simulink model "Carrier_Phase_Shift"  (R2021a)
settings: Solver=FixedStepAuto  StartTime=0.0  StopTime=0.05  FixedStep=1e-7  MaxStep=1e-7  RelTol=1e-6
InitFcn:
  | fsw=50e3;
  | ma=0.6;
  | ffund=100;
  | 
  | L1=63e-6;
  | L2=50e-6;
  | M=18e-6;
  | C1=12.2e-9;
  | C2=14.5e-9;
  | R=20;
  | 
  | sn3=C1*C2*M*R;
  | sd4=C1*C2*L1*L2+C1*C2*L1*M+C1*C2*L2*M;
  | sd3= C1*C2*L1*R+ C1*C2*M*R;
  | sd2= C1*L1+C2*L2+C1*M+C2*M;
  | sd1=C2*R;
  | sd0=1;
libraries: spsSeriesRLCBranchLib x9, spsDiodeLib x4, spsVoltageMeasurementLib x3, spsControlledVoltageSourceLib x1, spsCurrentMeasurementLib x1, dspsigops x1, spspowerguiLib x1
settings Model: Creator=enes_  LastModifiedBy=enes_
settings DataIOCC: SaveFormat=StructureWithTime  ReturnWorkspaceOutputs=off

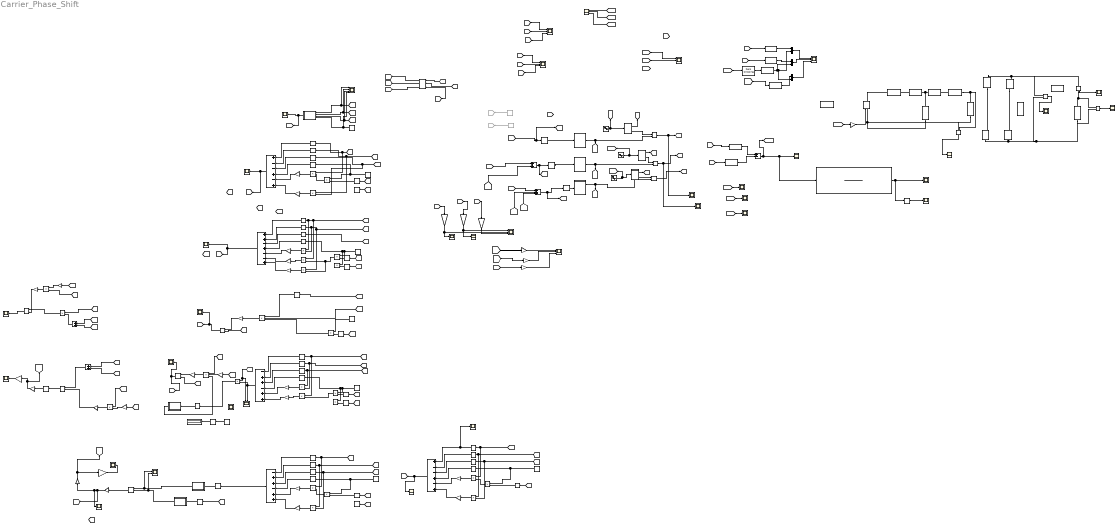
== system Carrier_Phase_Shift ==
  Abs : Abs
  Add : Sum  Inputs=+--+-+
  Add1 : Sum  Inputs=++-+--+
  Add2 : Sum  Inputs=-++-++
  Add3 : Sum
  Add4 : Sum
  Add5 : Sum
  Add6 : Sum  Inputs=+--+-+
  Add7 : Sum  Inputs=+++
  Add8 : Sum  Inputs=-++-++
  Atan : Trigonometry  Operator=atan
  Atan1 : Trigonometry  Operator=atan2
  Constant : Constant  Commented=on  Value=0
  Constant{1,3..8} (7 alike) : Constant  Value=0.95
  Constant2 : Constant  Commented=on  Value=pi
  Controlled Voltage Source : spsControlledVoltageSourceLib/Controlled Voltage Source  Initialize=on  Source_Type=AC  Amplitude=0  Phase=0  Frequency=0  Measurements=None
  Cos{,2,4,8..9} (5 alike) : Trigonometry  Operator=cos
  Cos{1,3,5..6,10} (5 alike) : Trigonometry
  Current Measurement : spsCurrentMeasurementLib/Current Measurement  PhasorSimulation=off  OutputType=Complex  PSBequivalent=0
  Data Type Conversion{,1..2,4..6} (6 alike) : DataTypeConversion
  Delay : Delay  DelayLength=1
  Delay1 : Delay  DelayLength=1
  Delay2 : Delay  DelayLength=1
  Diode{,1..3} (4 alike) : spsDiodeLib/Diode  Ron=0.001  Lon=0  Vf=0.8  IC=0  UseSnubber=0  Rs=500  Cs=250e-9  Measurements=on
  Display : Display
  Divide{,1,3..4} (4 alike) : Product  Inputs=*/
  Gain : Gain  Gain=100
  Gain10 : Gain  Gain=8
  Gain{9,12..13,23,28..30,33} (8 alike) : Gain  Gain=180/pi
  Gain{2..3,5..7,14..16,18,20,22,25,27,31..32,34} (16 alike) : Gain  Gain=2
  Gain17 : Gain  Gain=4
  Gain19 : Gain  Gain=4
  Gain21 : Gain  Gain=4
  Gain35 : Gain  Gain=-1
  Goto18 : Goto  Commented=on  GotoTag=CP_A
  Goto19 : Goto  Commented=on  GotoTag=CP_BA
  MATLAB Function : MATLAB Function  TreatAsAtomicUnit=on
  MATLAB Function1 : MATLAB Function  TreatAsAtomicUnit=on
  MATLAB Function2 : MATLAB Function  TreatAsAtomicUnit=on
  MATLAB Function3 : MATLAB Function  TreatAsAtomicUnit=on
  Mux : Mux  Inputs=2
  Mux1 : Mux  Inputs=2
  Mux2 : Mux  Inputs=2
  Product{,1..7,9..14,16..19,21..23,25..26} (23 alike) : Product
  Product15 : Product  Inputs=3
  Product8 : Product  Inputs=3
  Relational Operator : RelationalOperator  OutDataTypeStr=boolean  RndMeth=Simplest
  Relational Operator1 : RelationalOperator  OutDataTypeStr=boolean  RndMeth=Simplest
  Relational Operator2 : RelationalOperator  OutDataTypeStr=boolean  RndMeth=Simplest
  Scope{,8,27,29..30,38..39} (7 alike) : Scope  NumInputPorts=3
  Scope{1..7,9..14,16..22,25..26,28,31,33} (25 alike) : Scope
  Scope15 : Scope  NumInputPorts=4
  Scope23 : Scope  NumInputPorts=2
  Scope24 : Scope  NumInputPorts=2
  Scope32 : Scope  NumInputPorts=2
  Series RLC Branch : spsSeriesRLCBranchLib/Series RLC Branch  LConnTagsString=__new0  RConnTagsString=__new0  BranchType=C  Resistance=1  Inductance=1e-3  SetiL0=off  InitialCurrent=0  Capacitance=12.2e-9  Setx0=off  InitialVoltage=0  Measurements=None
  Series RLC Branch1 : spsSeriesRLCBranchLib/Series RLC Branch  LConnTagsString=__new0  RConnTagsString=__new0  BranchType=C  Resistance=1  Inductance=1e-3  SetiL0=off  InitialCurrent=0  Capacitance=14.5e-9  Setx0=off  InitialVoltage=0  Measurements=None
  Series RLC Branch2 : spsSeriesRLCBranchLib/Series RLC Branch  LConnTagsString=__new0  RConnTagsString=__new0  BranchType=L  Resistance=1  Inductance=63e-6  SetiL0=off  InitialCurrent=0  Capacitance=1e-6  Setx0=off  InitialVoltage=0  Measurements=None
  Series RLC Branch3 : spsSeriesRLCBranchLib/Series RLC Branch  LConnTagsString=__new0  RConnTagsString=__new0  BranchType=L  Resistance=1  Inductance=18e-6  SetiL0=off  InitialCurrent=0  Capacitance=1e-6  Setx0=off  InitialVoltage=0  Measurements=None
  Series RLC Branch4 : spsSeriesRLCBranchLib/Series RLC Branch  LConnTagsString=__new0  RConnTagsString=__new0  BranchType=L  Resistance=1  Inductance=50e-6  SetiL0=off  InitialCurrent=0  Capacitance=1e-6  Setx0=off  InitialVoltage=0  Measurements=None
  Series RLC Branch5 : spsSeriesRLCBranchLib/Series RLC Branch  LConnTagsString=__new0  RConnTagsString=__new0  BranchType=C  Resistance=1  Inductance=1e-3  SetiL0=off  InitialCurrent=0  Capacitance=100e-6  Setx0=off  InitialVoltage=0  Measurements=None
  Series RLC Branch6 : spsSeriesRLCBranchLib/Series RLC Branch  LConnTagsString=__new0  RConnTagsString=__new0  BranchType=L  Resistance=1  Inductance=500e-6  SetiL0=off  InitialCurrent=0  Capacitance=14.5e-9  Setx0=off  InitialVoltage=0  Measurements=None
  Series RLC Branch7 : spsSeriesRLCBranchLib/Series RLC Branch  LConnTagsString=__new0  RConnTagsString=__new0  BranchType=R  Resistance=40  Inductance=5e-3  SetiL0=off  InitialCurrent=0  Capacitance=1e-6  Setx0=off  InitialVoltage=0  Measurements=None
  Series RLC Branch8 : spsSeriesRLCBranchLib/Series RLC Branch  LConnTagsString=__new0  RConnTagsString=__new0  BranchType=R  Resistance=40  Inductance=5e-3  SetiL0=off  InitialCurrent=0  Capacitance=1e-6  Setx0=off  InitialVoltage=0  Measurements=None
  Sine Wave : Sin  Amplitude=ma  Frequency=2*pi*ffund  SampleTime=0
  Sine Wave1 : Sin  Amplitude=ma  Frequency=2*pi*ffund  Phase=2*pi/3  SampleTime=0
  Sine Wave2 : Sin  Amplitude=ma  Frequency=2*pi*ffund  Phase=-2*pi/3  SampleTime=0
  Sqrt{,1..3} (4 alike) : Sqrt  OutputSignalType=real  SaturateOnIntegerOverflow=on
  Square{,1..20} (21 alike) : Math  Operator=square  SaturateOnIntegerOverflow=on
  Subsystem2 : Subsystem
  Subsystem3 : Subsystem
  Subsystem4 : Subsystem
  Subsystem5 : Subsystem
  Subtract : Sum  Inputs=+-
  Transfer Fcn : TransferFcn  Numerator=[sn3 0 0 0]  Denominator=[sd4 sd3 sd2 sd1 sd0]
  Triangle Generator-A : Subsystem
  Triangle Generator-A1 : Subsystem
  Triangle Generator-A2 : Subsystem
  Voltage Measurement : spsVoltageMeasurementLib/Voltage Measurement  PhasorSimulation=off  OutputType=Complex  PSBequivalent=0
  Voltage Measurement1 : spsVoltageMeasurementLib/Voltage Measurement  PhasorSimulation=off  OutputType=Complex  PSBequivalent=0
  Voltage Measurement2 : spsVoltageMeasurementLib/Voltage Measurement  PhasorSimulation=off  OutputType=Complex  PSBequivalent=0
  Zero Crossing2 : dspsigops/Zero Crossing  InputProcessing=Columns as channels (frame based)
      settings: SourceProductBaseCode=DS
  Zero3 : Constant  Value=1e-15  OutDataTypeStr=Inherit: Inherit via back propagation
  powergui : spspowerguiLib/powergui  Priority=1  SimulationMode=Continuous  SampleTime=50e-6  frequency=60  Iterations=50  frequencyindice=0  Pbase=100e6  ErrMax=1e-4  UnitsV=kV  UnitsW=MW  buscounter=0  FunctionMessages=off  echomessages=off  EnableUseOfTLC=off  CurrentSourceSwitches=off  DisableSnubberDevices=off  DisableRonSwitches=off  DisableVfSwitches=off  DisplayEquations=off  AutomaticDiscreteSolvers=off  SolverType=Tustin/Backward Euler (TBE)  Interpol=off  ExternalGateDelay=off  methode=off  Ts=100  x0status=blocks  SPID=on  SwTol=0  HookPort=off  NonlinearTolerance=1e-4  nMaxIteration=100  ContinueOnMaxIteration=off  RestoreLinks=warning  ResistiveCurrentMeasurement=off  Frange=[0:2:500]  Ylog=off  Xlog=on  ShowGrid=off  save=off  variable=ZData  structure=0  ZoomFFT=off  StartTime=0.0  cycles=1  DisplayStyle=1  fundamental=60  FreqAxis=off  MaxFrequency=1000  frequencyindicesteady=1  RmsSteady=1  display=off
  wires:
  Triangle Generator-A2/1(Carrier) -> [C_C], Relational Operator2/2
  Relational Operator1/1 -> Scope7/1, [PWMB]
  Data Type Conversion/1 -> Subtract/1
  Data Type Conversion1/1 -> Subtract/2
  Delay1/1 -> Triangle Generator-A1/1(Phase)
  Delay2/1 -> Triangle Generator-A2/1(Phase)
  Add3/1 -> Delay1/1, [CP_B]
  Subtract/1 -> [PWMAB], Transfer Fcn/1, Scope2/1
  Delay/1 -> Triangle Generator-A/1(Phase)
  Gain12/1 -> Scope17/1, Scope27/1
  Gain13/1 -> Scope16/1, Scope27/2
  Subsystem4/2(Out2) -> Relational Operator2/1
  [DA] -> Scope29/1
  [DB] -> Scope29/2
  [Phase] -> Scope29/3
  [SB] -> Scope30/2
  [Phase] -> Scope30/3
  [SA] -> Scope30/1
  Triangle Generator-A/1(Carrier) -> Relational Operator/2, [C_A]
  Zero Crossing2/1 -> Data Type Conversion6/1
  [alpha] -> Add3/2
  [phi] -> Add3/1
  [CP_B] -> Gain13/1
  [CP_A] -> Gain12/1
  Subsystem2/1(Out1) -> [DA]
  Subsystem2/2(Out2) -> Relational Operator/1
  Triangle Generator-A1/1(Carrier) -> Relational Operator1/2, [C_B]
  Sine Wave1/1 -> [R_B], Subsystem3/1(In1)
  Subsystem3/1(Out1) -> [DB]
  Subsystem3/2(Out2) -> Relational Operator1/1
  Sine Wave/1 -> Subsystem2/1(In1), [R_A]
  [PWMA] -> Data Type Conversion4/1
  Mux/1 -> Scope39/1
  Mux1/1 -> Scope39/2
  Data Type Conversion4/1 -> Mux/1
  [PWMB] -> Data Type Conversion5/1
  Data Type Conversion5/1 -> Mux1/1
  Data Type Conversion6/1 -> Mux1/2, Mux2/2, Mux/2
  Relational Operator/1 -> Scope6/1, [PWMA]
  Relational Operator2/1 -> [PWMC]
  [PWMA] -> Data Type Conversion/1
  [PWMB] -> Data Type Conversion1/1
  [PWMAB] -> Data Type Conversion2/1
  Mux2/1 -> Scope39/3
  Data Type Conversion2/1 -> Mux2/1
  [C_A] -> Zero Crossing2/1
  [C_A] -> Scope/1
  [C_B] -> Scope/2
  [PWMAB] -> Gain/1
  Gain/1 -> Controlled Voltage Source/1
  Voltage Measurement/1 -> Scope1/1
  Voltage Measurement1/1 -> Scope3/1
  Current Measurement/1 -> Scope4/1
  Voltage Measurement2/1 -> Scope5/1
  [R_B] -> Scope38/2
  [R_C] -> Scope38/3
  [R_A] -> Scope38/1
  Constant/1 -> Goto18/1
  Constant2/1 -> Goto19/1
  [C_A] -> Scope9/1
  [C_B] -> Scope10/1
  [C_C] -> Scope11/1
  Transfer Fcn/1 -> Abs/1, Scope12/1
  Abs/1 -> Scope13/1
  Sine Wave2/1 -> [R_C], Subsystem4/1(In1)
  Subsystem4/1(Out1) -> [DC]
  Subsystem5/2(Out2) -> [SB]
  [DA] -> Subsystem5/1(In1)
  [DB] -> Subsystem5/2(In2)
  Subsystem5/1(Out1) -> [SA]
  Subsystem5/3(Out3) -> [SC]
  [DC] -> Subsystem5/3(In3)
  [SB] -> Scope15/2, MATLAB Function/2(SB)
  Constant4/1 -> Scope15/4, MATLAB Function/4(SABC)
  [SA] -> Scope15/1, MATLAB Function/1(SA)
  [SC] -> Scope15/3, MATLAB Function/3(SC)
  [phi] -> [CP_A], Delay/1
  MATLAB Function/1(phi) -> [phi], Scope14/1
  [SC] -> Product2/2, Square2/1
  Constant1/1 -> Product1/1, Square3/1
  [SB] -> Product2/1, Square1/1
  [SA] -> Product/1, Square/1
  [phi] -> Cos/1
  [phi] -> Cos1/1
  Cos/1 -> Product1/2
  Product1/1 -> Product/2
  Product/1 -> Gain2/1
  Product2/1 -> Gain3/1
  Square/1 -> Add/1
  Square1/1 -> Add/2
  Square2/1 -> Add/3
  Square3/1 -> Add/4
  Gain2/1 -> Add/5
  Gain3/1 -> Add/6
  Add/1 -> [sigma4], Scope18/1
  Product3/1 -> Gain5/1
  Square5/1 -> Add1/2
  Product5/1 -> Gain6/1
  Square4/1 -> Add1/1
  [phi] -> Cos3/1
  Square7/1 -> Add1/4
  Square6/1 -> Add1/3
  [SC] -> Square6/1
  [SB] -> Product3/2, Square5/1, Product5/1
  [phi] -> Cos2/1
  Gain5/1 -> Add1/5
  [SA] -> Product3/1, Square4/1, Product4/1
  Cos2/1 -> Product6/2
  Cos3/1 -> Product7/2
  Constant3/1 -> Product6/1, Product7/1, Square7/1
  Product6/1 -> Product5/2, Product4/2
  Product4/1 -> Gain7/1
  Gain7/1 -> Add1/6
  Gain6/1 -> Add1/7
  Add1/1 -> Scope19/1, [sigma3]
  Cos5/1 -> Product12/2
  [SC] -> Product8/2
  [SB] -> Square9/1
  [phi] -> Cos5/1
  Constant5/1 -> Product12/1
  Square9/1 -> Product8/1
  Product12/1 -> Product8/3
  Product8/1 -> Gain10/1
  Gain16/1 -> Add2/6
  Cos6/1 -> Product14/2
  Product13/1 -> Product10/2
  Cos4/1 -> Product13/2
  Product10/1 -> Gain16/1
  Gain14/1 -> Add2/5
  [SB] -> Product9/2, Square10/1
  [phi] -> Cos4/1
  [phi] -> Cos6/1
  [SA] -> Square8/1, Product10/1
  Square12/1 -> Add2/4
  Constant6/1 -> Product13/1, Product14/1, Square12/1
  Square8/1 -> Add2/1
  Product9/1 -> Gain14/1
  Square10/1 -> Add2/2
  Square11/1 -> Add2/3
  [SC] -> Product9/1, Square11/1
  Add2/1 -> Product11/2, Scope23/2
  [sigma4] -> Scope23/1, Product11/1
  [SB] -> Gain15/1
  Gain15/1 -> Product15/2
  [SC] -> Product15/1
  Product15/1 -> Gain17/1
  [sigma1] -> Add4/1
  [sigma2] -> Add4/2
  [sigma4] -> Product16/1
  Add4/1 -> Product16/2
  [SB] -> Gain18/1
  Gain18/1 -> Product17/1
  [SC] -> Product17/2
  Product17/1 -> Gain19/1
  Product16/1 -> Divide/1
  Gain19/1 -> Divide/2
  Divide/1 -> Scope25/1
  Product11/1 -> Sqrt/1
  Zero3/1 -> Sqrt1/1
  Sqrt1/1 -> Display/1
  Sqrt/1 -> MATLAB Function1/1(u)
  MATLAB Function1/1(y) -> Product15/3
  [SB] -> Gain20/1
  Product18/1 -> Gain21/1
  [SC] -> Product18/1
  Gain20/1 -> Product18/2
  [sigma1] -> Add5/1
  [sigma2] -> Add5/2
  Add5/1 -> Divide1/1
  Gain21/1 -> Divide1/2
  Divide1/1 -> Atan/1
  Atan/1 -> Gain22/1
  Gain22/1 -> [alpha], Gain23/1
  Gain23/1 -> Scope22/1
  [CP_C] -> Gain28/1
  Gain28/1 -> Scope27/3
  Add7/1 -> [CP_C], Delay2/1
  [beta] -> Add7/3
  [alpha] -> Add7/2
  [phi] -> Add7/1
  [alpha] -> Gain9/1
  Gain9/1 -> Scope8/1
  [beta] -> Gain29/1
  Gain29/1 -> Scope8/2
  Gain30/1 -> Scope8/3
  [phi] -> Gain30/1
  Gain10/1 -> Divide3/1
  Divide3/1 -> Scope20/1, [sigma2]
  [sigma3] -> Divide3/2
  Gain17/1 -> Divide4/1
  Divide4/1 -> [sigma1], Scope21/1
  [sigma3] -> Divide4/2
  Sqrt2/1 -> MATLAB Function2/1(u)
  Add8/1 -> Sqrt2/1
  [SA] -> Square17/1, Product23/1
  Product23/1 -> Gain31/1
  [phi] -> Cos9/1
  Square19/1 -> Add8/3
  Product26/1 -> Gain32/1
  Product25/1 -> Product23/2
  [SB] -> Product26/1, Square18/1
  Square18/1 -> Add8/2
  [phi] -> Cos10/1
  Gain32/1 -> Add8/6
  Cos9/1 -> Product25/2
  [SC] -> Product26/2, Square19/1
  Constant8/1 -> Product25/1, Square20/1
  Square20/1 -> Add8/4
  Gain31/1 -> Add8/5
  Square17/1 -> Add8/1
  Square13/1 -> Scope33/1, Add6/1
  Square16/1 -> Add6/4
  Gain25/1 -> Add6/5
  Constant7/1 -> Product21/1, Square16/1
  [SC] -> Product22/2, Square15/1
  Gain27/1 -> Add6/6
  Cos8/1 -> Product21/2
  Product22/1 -> Gain27/1
  Square15/1 -> Add6/3
  [SB] -> Product22/1, Square14/1
  Product19/1 -> Gain25/1
  [phi] -> Cos8/1
  Square14/1 -> Add6/2
  [SA] -> Square13/1, Product19/1
  Product21/1 -> Product19/2
  Gain33/1 -> Scope26/1
  Atan1/1 -> Gain34/1
  Add6/1 -> Scope28/1, [sigma6]
  Gain34/1 -> [sigma5], Gain35/1, Scope31/1
  Gain35/1 -> [beta], Gain33/1
  MATLAB Function2/1(y) -> Scope32/1, Atan1/1
  Sqrt3/1 -> MATLAB Function3/1(u)
  [sigma6] -> Sqrt3/1
  MATLAB Function3/1(y) -> Scope32/2, Atan1/2
  connections:
  Series RLC Branch/LConn1 -- Controlled Voltage Source/RConn1
  Series RLC Branch2/LConn1 -- Series RLC Branch/RConn1
  Series RLC Branch3/LConn1 -- Series RLC Branch4/LConn1 -- Series RLC Branch2/RConn1
  Series RLC Branch1/LConn1 -- Series RLC Branch4/RConn1
  Series RLC Branch1/RConn1 -- Series RLC Branch8/LConn1 -- Voltage Measurement2/LConn1
  Series RLC Branch3/RConn1 -- Series RLC Branch8/RConn1 -- Voltage Measurement2/LConn2 -- Controlled Voltage Source/LConn1
  Diode/RConn1 -- Current Measurement/LConn1 -- Voltage Measurement1/LConn1 -- Diode2/RConn1
  Diode1/LConn1 -- Voltage Measurement1/LConn2 -- Voltage Measurement/LConn2 -- Series RLC Branch7/RConn1 -- Diode3/LConn1
  Voltage Measurement/LConn1 -- Current Measurement/RConn1 -- Series RLC Branch7/LConn1
  Diode/LConn1 -- Diode1/RConn1
  Diode2/LConn1 -- Diode3/RConn1

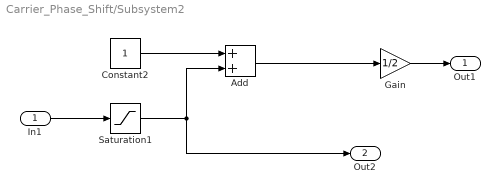
== system Carrier_Phase_Shift/Subsystem2 ==
  In1 : Inport
  Add : Sum
  Constant2 : Constant
  Gain : Gain  Gain=1/2
  Saturation1 : Saturate  UpperLimit=1  LowerLimit=-1
  Out1 : Outport
  Out2 : Outport  Port=2
  wires:
  Constant2/1 -> Add/1
  Add/1 -> Gain/1
  Gain/1 -> Out1/1
  In1/1 -> Saturation1/1
  Saturation1/1 -> Out2/1, Add/2

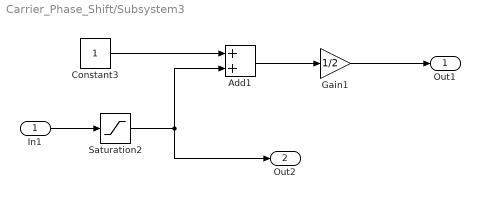
== system Carrier_Phase_Shift/Subsystem3 ==
  In1 : Inport
  Add1 : Sum
  Constant3 : Constant
  Gain1 : Gain  Gain=1/2
  Saturation2 : Saturate  UpperLimit=1  LowerLimit=-1
  Out1 : Outport
  Out2 : Outport  Port=2
  wires:
  Saturation2/1 -> Out2/1, Add1/2
  In1/1 -> Saturation2/1
  Constant3/1 -> Add1/1
  Add1/1 -> Gain1/1
  Gain1/1 -> Out1/1

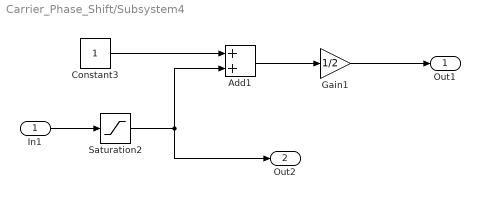
== system Carrier_Phase_Shift/Subsystem4 ==
  In1 : Inport
  Add1 : Sum
  Constant3 : Constant
  Gain1 : Gain  Gain=1/2
  Saturation2 : Saturate  UpperLimit=1  LowerLimit=-1
  Out1 : Outport
  Out2 : Outport  Port=2
  wires:
  Saturation2/1 -> Out2/1, Add1/2
  In1/1 -> Saturation2/1
  Constant3/1 -> Add1/1
  Add1/1 -> Gain1/1
  Gain1/1 -> Out1/1

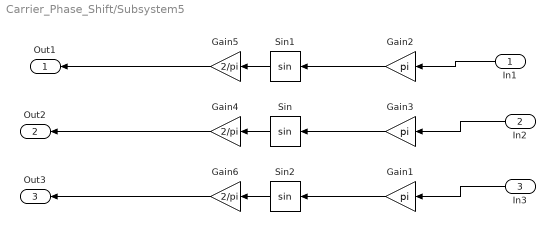
== system Carrier_Phase_Shift/Subsystem5 ==
  In1 : Inport
  In2 : Inport  Port=2
  In3 : Inport  Port=3
  Gain1 : Gain  Gain=pi
  Gain2 : Gain  Gain=pi
  Gain3 : Gain  Gain=pi
  Gain4 : Gain  Gain=2/pi
  Gain5 : Gain  Gain=2/pi
  Gain6 : Gain  Gain=2/pi
  Sin : Trigonometry
  Sin1 : Trigonometry
  Sin2 : Trigonometry
  Out1 : Outport
  Out2 : Outport  Port=2
  Out3 : Outport  Port=3
  wires:
  Gain4/1 -> Out2/1
  Gain3/1 -> Sin/1
  Gain2/1 -> Sin1/1
  Sin1/1 -> Gain5/1
  Sin/1 -> Gain4/1
  In1/1 -> Gain2/1
  In2/1 -> Gain3/1
  Gain5/1 -> Out1/1
  Gain6/1 -> Out3/1
  In3/1 -> Gain1/1
  Sin2/1 -> Gain6/1
  Gain1/1 -> Sin2/1

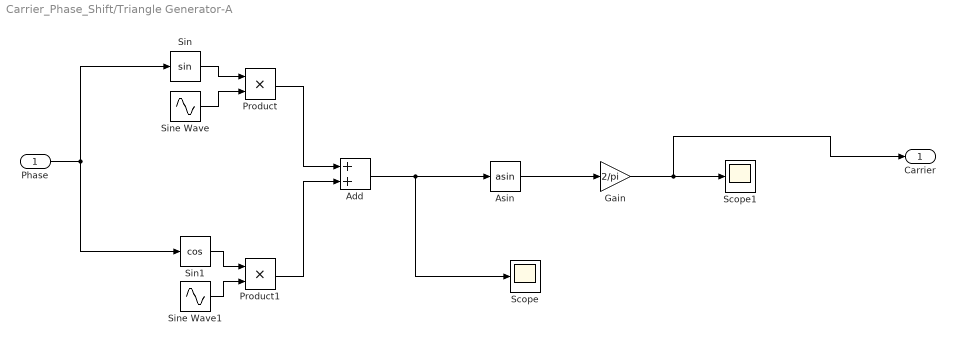
== system Carrier_Phase_Shift/Triangle Generator-A ==
  Phase : Inport
  Add : Sum
  Asin : Trigonometry  Operator=asin
  Gain : Gain  Gain=2/pi
  Product : Product
  Product1 : Product
  Scope : Scope
  Scope1 : Scope
  Sin : Trigonometry
  Sin1 : Trigonometry  Operator=cos
  Sine Wave : Sin  Frequency=2*pi*fsw  SampleTime=0
  Sine Wave1 : Sin  Frequency=2*pi*fsw  Phase=-pi/2  SampleTime=0
  Carrier : Outport
  wires:
  Sin/1 -> Product/1
  Sine Wave/1 -> Product/2
  Phase/1 -> Sin1/1, Sin/1
  Product/1 -> Add/1
  Asin/1 -> Gain/1
  Gain/1 -> Carrier/1, Scope1/1
  Sine Wave1/1 -> Product1/2
  Product1/1 -> Add/2
  Add/1 -> Asin/1, Scope/1
  Sin1/1 -> Product1/1

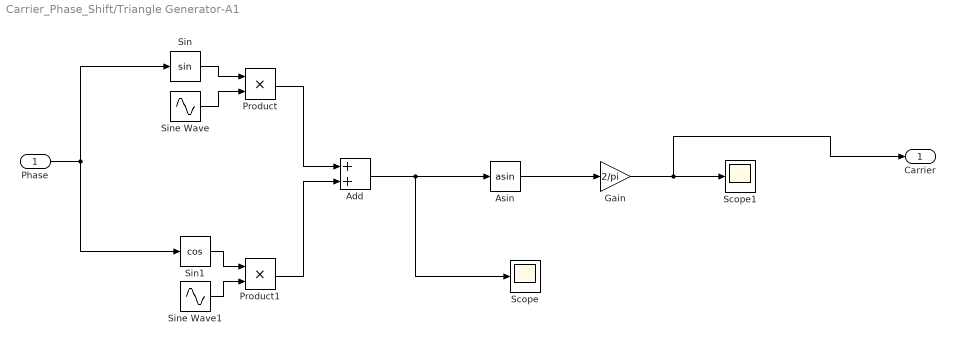
== system Carrier_Phase_Shift/Triangle Generator-A1 ==
  Phase : Inport
  Add : Sum
  Asin : Trigonometry  Operator=asin
  Gain : Gain  Gain=2/pi
  Product : Product
  Product1 : Product
  Scope : Scope
  Scope1 : Scope
  Sin : Trigonometry
  Sin1 : Trigonometry  Operator=cos
  Sine Wave : Sin  Frequency=2*pi*fsw  SampleTime=0
  Sine Wave1 : Sin  Frequency=2*pi*fsw  Phase=-pi/2  SampleTime=0
  Carrier : Outport
  wires:
  Sin/1 -> Product/1
  Sine Wave/1 -> Product/2
  Phase/1 -> Sin1/1, Sin/1
  Product/1 -> Add/1
  Asin/1 -> Gain/1
  Gain/1 -> Carrier/1, Scope1/1
  Sine Wave1/1 -> Product1/2
  Product1/1 -> Add/2
  Add/1 -> Asin/1, Scope/1
  Sin1/1 -> Product1/1

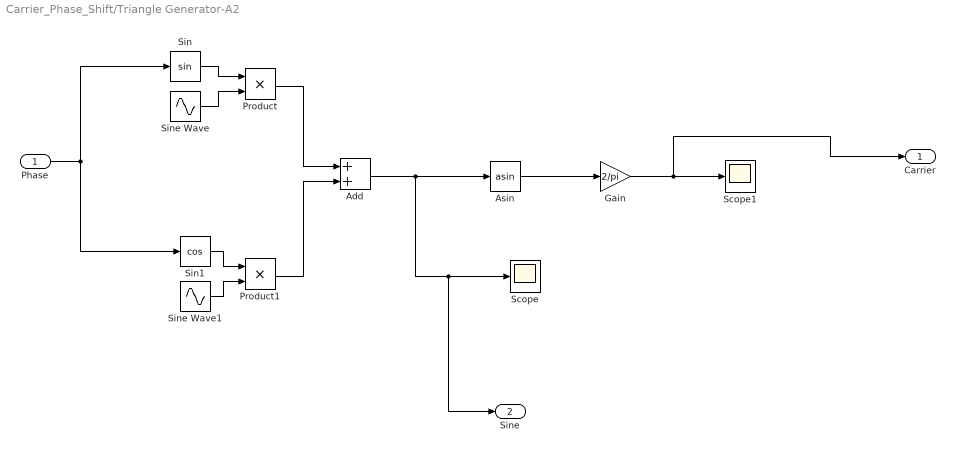
== system Carrier_Phase_Shift/Triangle Generator-A2 ==
  Phase : Inport
  Add : Sum
  Asin : Trigonometry  Operator=asin
  Gain : Gain  Gain=2/pi
  Product : Product
  Product1 : Product
  Scope : Scope
  Scope1 : Scope
  Sin : Trigonometry
  Sin1 : Trigonometry  Operator=cos
  Sine Wave : Sin  Frequency=2*pi*fsw  SampleTime=0
  Sine Wave1 : Sin  Frequency=2*pi*fsw  Phase=-pi/2  SampleTime=0
  Carrier : Outport
  Sine : Outport  Port=2
  wires:
  Sin/1 -> Product/1
  Sine Wave/1 -> Product/2
  Phase/1 -> Sin1/1, Sin/1
  Product/1 -> Add/1
  Asin/1 -> Gain/1
  Gain/1 -> Carrier/1, Scope1/1
  Sine Wave1/1 -> Product1/2
  Product1/1 -> Add/2
  Add/1 -> Asin/1, Sine/1, Scope/1
  Sin1/1 -> Product1/1

== matlab function Carrier_Phase_Shift/MATLAB Function1 ==
  data: u input; y output
function y = fcn(u)

if isnan(u)
    y=0;
else
y = u;
end

== matlab function Carrier_Phase_Shift/MATLAB Function ==
  data: SA input; phi output; SB input; SC input; SABC input
function phi = fcn(SA, SB, SC, SABC)

if SABC < SA- abs(SB-SC)
    phi=0;
elseif SABC > SA + abs(SB-SC)
        phi=0;   
else
   phi=acos((SA^2-(SB-SC)^2+SABC^2)/(SA*SABC));
   
end

== matlab function Carrier_Phase_Shift/MATLAB Function2 ==
  data: u input; y output
function y = fcn(u)

if isnan(u)
    y=0;
else
y = u;
end

== matlab function Carrier_Phase_Shift/MATLAB Function3 ==
  data: u input; y output
function y = fcn(u)

if isnan(u)
    y=0;
else
y = u;
end
